simulink model "Simu_Hochpass"  (R2015b)
settings: Solver=FixedStepAuto  StartTime=0.0  StopTime=10.0  RelTol=1e-3
libraries: simulink x3
settings Model: Creator=Wolfgang  LastModifiedBy=Wolfgang

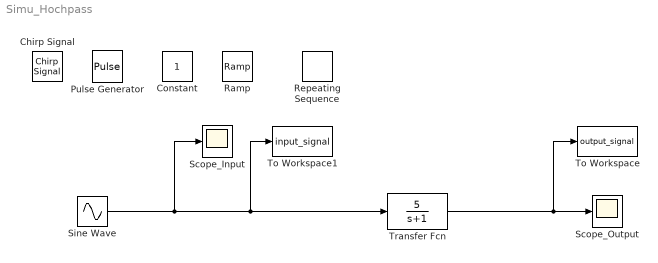
== system Simu_Hochpass ==
  Chirp Signal : simulink/Sources/Chirp Signal  f1=1  T=10  f2=0.001
  Constant : Constant
  Pulse Generator : DiscretePulseGenerator  PulseType=Time based  PulseWidth=5
  Ramp : simulink/Sources/Ramp  slope=1  start=0  X0=0
  Repeating Sequence : simulink/Sources/Repeating Sequence  rep_seq_t=[0 2]  rep_seq_y=[0 2]
  Scope_Input : Scope
  Scope_Output : Scope
  Sine Wave : Sin  SampleTime=0
  To Workspace : ToWorkspace  VariableName=output_signal  SampleTime=-1
  To Workspace1 : ToWorkspace  VariableName=input_signal  SampleTime=-1
  Transfer Fcn : TransferFcn  Numerator=[5]  Denominator=[1 1]
  wires:
  Sine Wave/1 -> Transfer Fcn/1, To Workspace1/1, Scope_Input/1
  Transfer Fcn/1 -> To Workspace/1, Scope_Output/1
